simulink model "foc_qep_host"  (R2025b)
settings: Solver=FixedStepDiscrete  StartTime=0.0  StopTime=Inf  RelTol=1e-3
undefined symbols (not defined in the file or in its folder): pmsm
libraries: instrumentseriallib x3

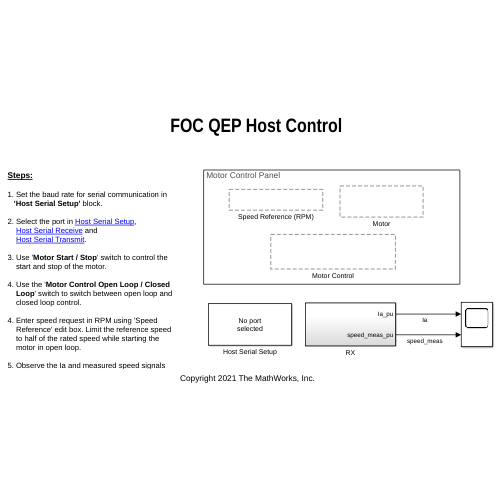
[thumbnail: Simulink's stored preview of the top-level diagram]
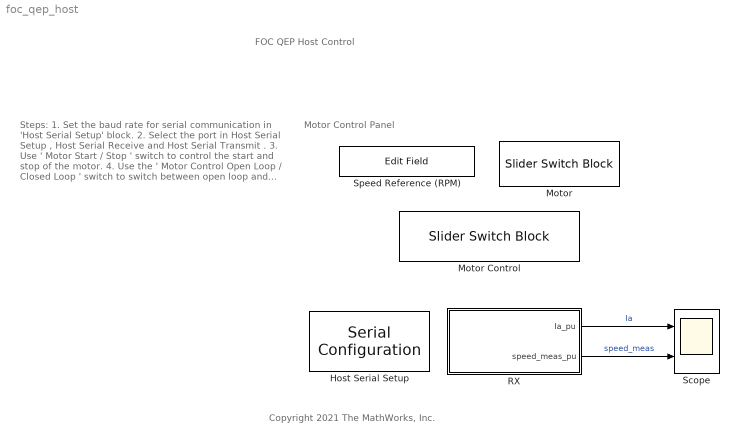
== system foc_qep_host ==
  note: FOC QEP Host Control
  note: Motor Control Panel
  note: Steps:
      |
      | 1. Set the baud rate for serial communication in
      | 'Host Serial Setup' block.
      |
      | 2. Select the port in Host Serial Setup ,
      | Host Serial Receive and
      | Host Serial Transmit .
      |
      | 3. Use ' Motor Start / Stop ' switch to control the
      | start and stop of the motor.
      |
      | 4. Use the ' Motor Control Open Loop / Closed
      | Loop ' switch to switch between open loop and
      | closed loop control.
      |
      | 4. Enter speed request in RPM using 'Speed
      | Reference' edit box. Limit the reference speed
      | to half of the rated speed while starting the
      | motor in open loop.
      |
      | 5. Observe the Ia and measured speed signals on the scope.
  note: Copyright 2021 The MathWorks, Inc.
  Host Serial Setup : instrumentseriallib/Serial Configuration  Priority=-99  PortSel=<Select a port...>  Port=<Select a port...>  ComPort=<Select a port...>  BaudRate=4000000  DataBits=8  Parity=none  StopBits=1  ByteOrder=little-endian  FlowControl=none  Timeout=2.0  SimulateUsing=Interpreted execution  BlockInModel=on  aMode=5
  Motor : SliderSwitchBlock  LabelPosition=Hide
  Motor Control : SliderSwitchBlock  LabelPosition=Hide
  RX : Subsystem
  Scope : Scope  NumInputPorts=2
  Speed Reference (RPM) : EditField  LabelPosition=Hide  ShowInitialText=on  Alignment=Center
  wires:
  RX/1(Ia_pu) -> Scope/1  "Ia"
  RX/2(speed_meas_pu) -> Scope/2  "speed_meas"

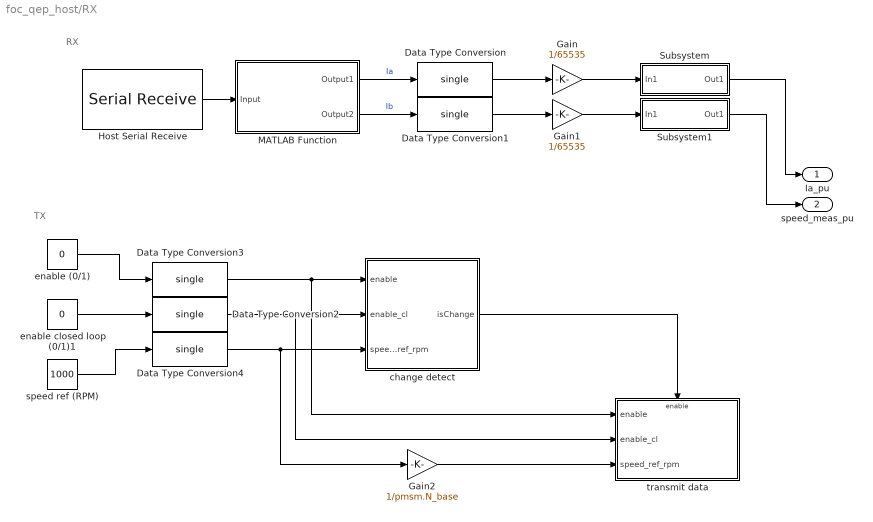
== system foc_qep_host/RX ==
  note: TX
  note: RX
  Data Type Conversion{,1..4} (5 alike) : DataTypeConversion  OutDataTypeStr=single  SaturateOnIntegerOverflow=off  RndMeth=Floor
  Gain : Gain  Gain=1/65535  OutDataTypeStr=single
  Gain1 : Gain  Gain=1/65535  OutDataTypeStr=single
  Gain2 : Gain  Gain=1/pmsm.N_base  OutDataTypeStr=single
  Host Serial Receive : instrumentseriallib/Serial Receive  PortSel=<Select a port...>  Port=<Select a port...>  ComPort=<Select a port...>  DataType=uint16  SaveDataType=uint8  ToggleHeader=on  Header='ss'  ToggleDataSize=on  DataSize=[200 2]  ToggleTerminator=on  Terminator=Custom terminator  CustomTerminator='ee'  InputFormat=Row major  EnableBlockingMode=on  ActionDataUnavailable=Output custom value  ActionWhenDataUnavailable=Output custom value  CustomValue=4000  SampleTime=200 * 50e-6  SimulateUsing=Interpreted execution  BlockInModel=on  aMode=5  LibraryInUse=instrumentlib
  MATLAB Function : MATLAB Function  TreatAsAtomicUnit=on
  Subsystem : Subsystem
  Subsystem1 : Subsystem
  change detect : Subsystem
  enable (0/1) : Constant  Value=0  OutDataTypeStr=boolean  SampleTime=-1
  enable closed loop (0/1)1 : Constant  Value=0  OutDataTypeStr=boolean  SampleTime=-1
  speed ref (RPM) : Constant  Value=1000  OutDataTypeStr=single  SampleTime=-1
  transmit data : Subsystem  TreatAsAtomicUnit=on
  Ia_pu : Outport
  speed_meas_pu : Outport  Port=2
  wires:
  Subsystem/1(Out1) -> Ia_pu/1
  Subsystem1/1(Out1) -> speed_meas_pu/1
  Data Type Conversion/1 -> Gain/1
  Data Type Conversion1/1 -> Gain1/1
  Gain/1 -> Subsystem/1(In1)
  MATLAB Function/1(Output1) -> Data Type Conversion/1  "Ia"
  Gain1/1 -> Subsystem1/1(In1)
  Host Serial Receive/1 -> MATLAB Function/1(Input)
  MATLAB Function/2(Output2) -> Data Type Conversion1/1  "Ib"
  Gain2/1 -> transmit data/3(speed_ref_rpm)
  enable (0/1)/1 -> Data Type Conversion3/1
  Data Type Conversion2/1 -> transmit data/2(enable_cl), change detect/2(enable_cl)
  enable closed loop (0/1)1/1 -> Data Type Conversion2/1
  Data Type Conversion4/1 -> Gain2/1, change detect/3(speed_ref_rpm)
  Data Type Conversion3/1 -> transmit data/1(enable), change detect/1(enable)
  change detect/1(isChange) -> transmit data/Enable
  speed ref (RPM)/1 -> Data Type Conversion4/1

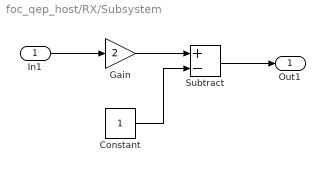
== system foc_qep_host/RX/Subsystem ==
  In1 : Inport
  Constant : Constant
  Gain : Gain  Gain=2
  Subtract : Sum  Inputs=+-
  Out1 : Outport
  wires:
  In1/1 -> Gain/1
  Gain/1 -> Subtract/1
  Subtract/1 -> Out1/1
  Constant/1 -> Subtract/2

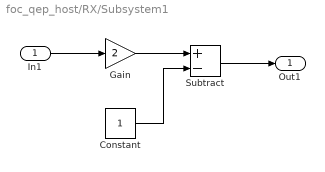
== system foc_qep_host/RX/Subsystem1 ==
  In1 : Inport
  Constant : Constant
  Gain : Gain  Gain=2
  Subtract : Sum  Inputs=+-
  Out1 : Outport
  wires:
  In1/1 -> Gain/1
  Gain/1 -> Subtract/1
  Subtract/1 -> Out1/1
  Constant/1 -> Subtract/2

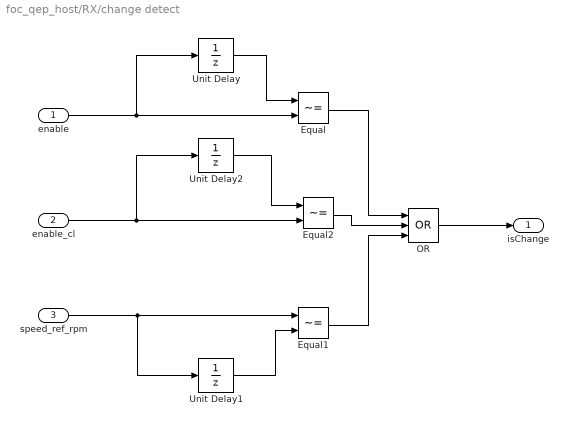
== system foc_qep_host/RX/change detect ==
  enable : Inport
  enable_cl : Inport  Port=2
  speed_ref_rpm : Inport  Port=3
  Equal : RelationalOperator  Operator=~=  OutDataTypeStr=boolean  RndMeth=Simplest  InputSameDT=off
  Equal1 : RelationalOperator  Operator=~=  OutDataTypeStr=boolean  RndMeth=Simplest  InputSameDT=off
  Equal2 : RelationalOperator  Operator=~=  OutDataTypeStr=boolean  RndMeth=Simplest  InputSameDT=off
  OR : Logic  Operator=OR  Inputs=3  AllPortsSameDT=off  OutDataTypeStr=boolean
  Unit Delay : UnitDelay  SampleTime=-1  HasFrameUpgradeWarning=on
  Unit Delay1 : UnitDelay  SampleTime=-1  HasFrameUpgradeWarning=on
  Unit Delay2 : UnitDelay  SampleTime=-1  HasFrameUpgradeWarning=on
  isChange : Outport
  wires:
  Unit Delay/1 -> Equal/1
  enable/1 -> Equal/2, Unit Delay/1
  speed_ref_rpm/1 -> Unit Delay1/1, Equal1/1
  Unit Delay1/1 -> Equal1/2
  OR/1 -> isChange/1
  Equal/1 -> OR/1
  Equal1/1 -> OR/3
  Equal2/1 -> OR/2
  enable_cl/1 -> Unit Delay2/1, Equal2/2
  Unit Delay2/1 -> Equal2/1

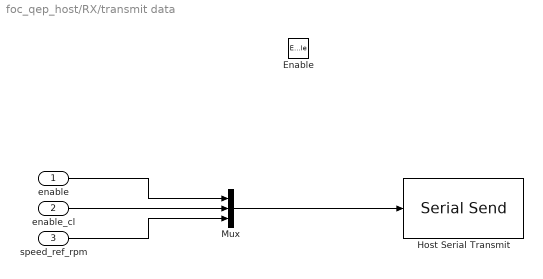
== system foc_qep_host/RX/transmit data ==
  enable : Inport
  enable_cl : Inport  Port=2
  speed_ref_rpm : Inport  Port=3
  Enable : EnablePort
  Host Serial Transmit : instrumentseriallib/Serial Send  PortSel=<Select a port...>  Port=<Select a port...>  ComPort=<Select a port...>  Header=[]  Terminator=<none>  CustomTerminator=[]  EnableBlockingMode=off  SimulateUsing=Interpreted execution  BlockInModel=off  aMode=5
  Mux : Mux  Inputs=3
  wires:
  enable/1 -> Mux/1
  Mux/1 -> Host Serial Transmit/1
  speed_ref_rpm/1 -> Mux/3
  enable_cl/1 -> Mux/2

== matlab function foc_qep_host/RX/MATLAB Function ==
function [ Output1, Output2] = unBuf(Input)

Output1 = Input(:, 1);
Output2 = Input(:, 2);
end
